simulink model "traal"  (R2019b)
settings: Solver=ode3  StartTime=0.0  StopTime=inf  RelTol=1e-3  EnableMultiTasking=on
undefined symbols (not defined in the file): Dist, Dist2, Ovrsht, Saved, trees
libraries: legoev3lib x15
settings Model: FPTRunName=Active  ExtModeTrigDuration=2  Creator=maarten  LastModifiedBy=Mohammed
settings SolverCC: PositivePriorityOrder=on
settings DataIOCC: LimitDataPoints=on  SaveFormat=Array
settings OptimizationCC: ExpressionDepthLimit=2147483647  LifeSpan=Inf  MaxStackSize=64
settings DebuggingCC: UnderspecifiedInitializationDetection=Classic  MergeDetectMultiDrivingBlocksExec=none  FcnCallInpInsideContextMsg=warning  AllowSymbolicDim=off  StateNameClashWarn=warning  SFUnexpectedBacktrackingDiag=warning  SFNoUnconditionalDefaultTransitionDiag=warning  SFExecutionAtInitializationDiag=none  ArithmeticOperatorsInVariantConditions=warning
settings HardwareCC: ProdBitPerPointer=32  ProdBitPerSizeT=32  ProdBitPerPtrDiffT=32  ProdLargestAtomicInteger=Long  ProdWordSize=32  ProdHWDeviceType=ARM Compatible->ARM 9  UseEmbeddedCoderFeatures=off  UseSimulinkCoderFeatures=off
settings ModelReferenceCC: PropagateSignalLabelsOutOfModel=off
settings SFSimCC: SimUseLocalCustomCode=off  CustomCodeUndefinedFunction=UseInterfaceOnly
settings RTWCC: SystemTargetFile=ert.tlc  HardwareBoard=LEGO MINDSTORMS EV3  TemplateMakefile=ert_default_tmf  GenerateReport=on  RTWVerbose=off  RTWUseLocalCustomCode=off  Toolchain=Sourcery G++ Lite v2009q3  BuildConfiguration=Faster Runs  LaunchReport=on
settings CodeAppCC: ForceParamTrailComments=on  OperatorAnnotations=on  MangleLength=10  StateflowObjectComments=on  MATLABSourceComments=on
settings ERTTargetCC: MultiwordLength=2048  ERTCustomFileBanners=off  SupportContinuousTime=on  SupportNonInlinedSFcns=on  RemoveResetFunc=off  SupportVariableSizeSignals=on  ModelStepFunctionPrototypeControlCompliant=off
settings ConfigComp: CovMetricSettings=dw  CovHtmlReporting=on  CovSaveCumulativeToWorkspaceVar=on  CovSaveSingleToWorkspaceVar=on  CovExternalEMLEnable=off  CovSFcnEnable=off

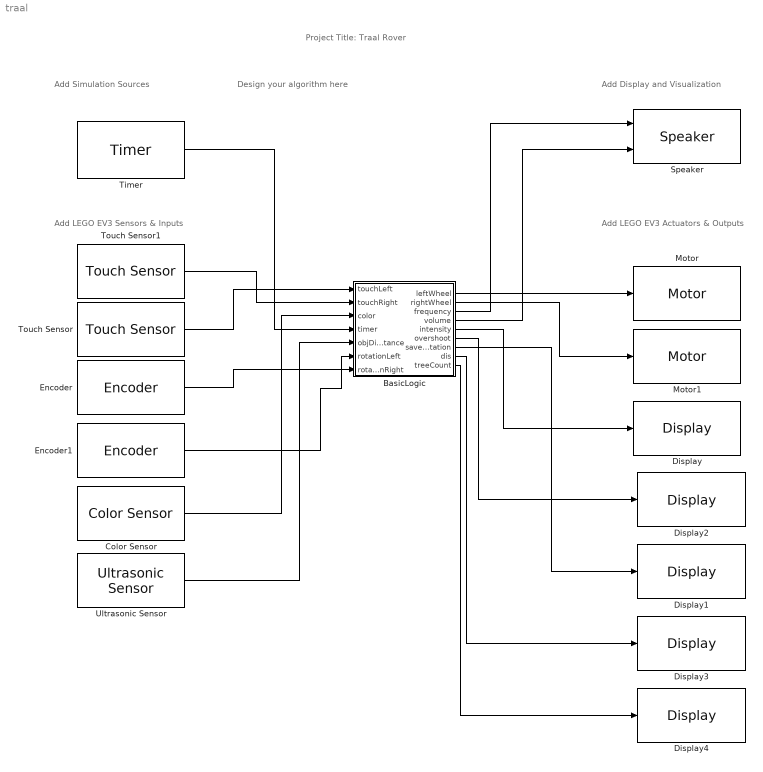
== system traal ==
  note: Project Title: Traal Rover
  note: Add LEGO EV3 Sensors & Inputs
  note: Add LEGO EV3 Actuators & Outputs
  note: Add Display and Visualization
  note: Design your algorithm here
  note: Add Simulation Sources
  BasicLogic : Stateflow chart  BlockKeywords=__PRM__SERIALIZED__DATA__:Stateflow Chart,Stateflow Diagram  TreatAsAtomicUnit=on
  Color Sensor : legoev3lib/Color Sensor  portNumber=3  mode=Reflected light intensity  sampleTime=0.1
      settings: SourceProductName=Simulink Support Package for LEGO MINDSTORMS EV3 Hardware  SourceProductBaseCode=LEGOEV3
  Display : legoev3lib/Display  slcdStr=Dist:  slcdLine=1  slcdFormat=Decimal
      settings: SourceProductName=Simulink Support Package for LEGO MINDSTORMS EV3 Hardware  SourceProductBaseCode=LEGOEV3
  Display1 : legoev3lib/Display  slcdStr=Saved:  slcdLine=3  slcdFormat=Decimal
      settings: SourceProductName=Simulink Support Package for LEGO MINDSTORMS EV3 Hardware  SourceProductBaseCode=LEGOEV3
  Display2 : legoev3lib/Display  slcdStr=Ovrsht:  slcdLine=2  slcdFormat=Decimal
      settings: SourceProductName=Simulink Support Package for LEGO MINDSTORMS EV3 Hardware  SourceProductBaseCode=LEGOEV3
  Display3 : legoev3lib/Display  slcdStr=Dist2:  slcdLine=4  slcdFormat=Decimal
      settings: SourceProductName=Simulink Support Package for LEGO MINDSTORMS EV3 Hardware  SourceProductBaseCode=LEGOEV3
  Display4 : legoev3lib/Display  slcdStr=trees:  slcdLine=5  slcdFormat=Decimal
      settings: SourceProductName=Simulink Support Package for LEGO MINDSTORMS EV3 Hardware  SourceProductBaseCode=LEGOEV3
  Encoder : legoev3lib/Encoder  portNumber=B  opMode=Reset by external signal  sampleTime=0.1
      settings: SourceProductName=Simulink Support Package for LEGO MINDSTORMS EV3 Hardware  SourceProductBaseCode=LEGOEV3
  Encoder1 : legoev3lib/Encoder  portNumber=C  opMode=Reset by external signal  sampleTime=0.1
      settings: SourceProductName=Simulink Support Package for LEGO MINDSTORMS EV3 Hardware  SourceProductBaseCode=LEGOEV3
  Motor : legoev3lib/Motor  sportNumber=C  sstopAction=Brake
  Motor1 : legoev3lib/Motor  sportNumber=B  sstopAction=Brake
  Speaker : legoev3lib/Speaker  sinputMode=Frequency and volume  sspeakerFreq=100  sspeakerVolume=50  sspeakerDuration=100
      settings: SourceProductName=Simulink Support Package for LEGO MINDSTORMS EV3 Hardware  SourceProductBaseCode=LEGOEV3
  Timer : legoev3lib/Timer  SampleTime=0.1
      settings: SourceProductName=Simulink Support Package for LEGO MINDSTORMS EV3 Hardware  SourceProductBaseCode=LEGOEV3
  Touch Sensor : legoev3lib/Touch Sensor  portNumber=1  sampleTime=0.1
      settings: SourceProductName=Simulink Support Package for LEGO MINDSTORMS EV3 Hardware  SourceProductBaseCode=LEGOEV3
  Touch Sensor1 : legoev3lib/Touch Sensor  portNumber=2  sampleTime=0.1
      settings: SourceProductName=Simulink Support Package for LEGO MINDSTORMS EV3 Hardware  SourceProductBaseCode=LEGOEV3
  Ultrasonic Sensor : legoev3lib/Ultrasonic Sensor  PortNumber=4  sampleTime=0.1
      settings: SourceProductName=Simulink Support Package for LEGO MINDSTORMS EV3 Hardware  SourceProductBaseCode=LEGOEV3
  wires:
  Touch Sensor/1 -> BasicLogic/1(touchLeft)
  BasicLogic/1(leftWheel) -> Motor/1
  BasicLogic/2(rightWheel) -> Motor1/1
  Touch Sensor1/1 -> BasicLogic/2(touchRight)
  Color Sensor/1 -> BasicLogic/3(color)
  Timer/1 -> BasicLogic/4(timer)
  BasicLogic/3(frequency) -> Speaker/1
  BasicLogic/4(volume) -> Speaker/2
  Ultrasonic Sensor/1 -> BasicLogic/5(objDistance)
  BasicLogic/5(intensity) -> Display/1
  Encoder/1 -> BasicLogic/7(rotationRight)
  Encoder1/1 -> BasicLogic/6(rotationLeft)
  BasicLogic/6(overshoot) -> Display2/1
  BasicLogic/7(savedRotation) -> Display1/1
  BasicLogic/8(dis) -> Display3/1
  BasicLogic/9(treeCount) -> Display4/1

== stateflow chart traal/BasicLogic ==
  state Master
    during:
    intensity = objDistance
    state ManualDriving
      during:
      dis = objDistance;
      state BothButtonsPressed
        entry:
        pressedTimer = timer
      state Forward
        entry: leftWheel = baseSpeed;
        rightWheel = baseSpeed;
        isStationary = false;
        fromAutonomous = false
      state Stationary
        entry: leftWheel = 0;
        rightWheel = 0;
        isStationary = true;
        fromAutonomous = false
      state ButtonsReleased
      state TurnLeft
        entry: leftWheel = 0;
        rightWheel = baseSpeed;
      state TurnRight
        entry: leftWheel = baseSpeed;
        rightWheel = 0;
      Forward -> (junction 31) [order 1] : [duration(touchLeft == 1) > 0.1]
      (default) -> Stationary
      Stationary -> BothButtonsPressed [order 3] : [touchLeft==1 && touchRight==1]
      Forward -> BothButtonsPressed [order 3] : [touchLeft==1 && touchRight==1]
      (junction 45) -> BothButtonsPressed : {isStationary = ~isStationary}
      BothButtonsPressed -> ButtonsReleased : [touchLeft==0 || touchRight==0]
      ButtonsReleased -> Stationary [order 3]
      ButtonsReleased -> Forward [order 2] : [timer - pressedTimer <= 1000 && isStationary]
      Stationary -> (junction 31) [order 2] : [duration(touchLeft == 1) > 0.2]
      (junction 31) -> TurnLeft
      Forward -> (junction 37) [order 2] : [duration(touchRight == 1) > 0.1]
      Stationary -> (junction 37) [order 1] : [duration(touchRight == 1) > 0.2]
      (junction 37) -> TurnRight
      TurnLeft -> (junction 45) : [touchLeft==0]
      TurnRight -> (junction 45) : [touchRight==0]
    state Finished
      entry:
      leftWheel = 0;
      rightWheel = 0;
      frequency = 4000;
      volume = 30;
      exit:
      frequency = 0;
      volume = 0;
    state Autonomous
      state GoToLine
        state goForward
          entry: leftWheel = 2 * baseSpeed;
          rightWheel = 2 * baseSpeed;
        state onLine
          entry:
          leftWheel = baseSpeed;
          rightWheel = baseSpeed;
        state BeyondLine
          entry: leftWheel = 0;
          rightWheel = 1.5 * baseSpeed;
        (default) -> goForward
        goForward -> onLine : [color < 25 ]
        onLine -> BeyondLine : [color > 20]
      state FollowLine
        during: dis = objDistance;
        state OnLine
          leftWheel = 1.5 * baseSpeed
          rightWheel = 1.5 * baseSpeed
          time = 0
        state startOnLine
          entry:
          leftWheel = baseSpeed
          rightWheel = baseSpeed
        state OffLineL
          entry:
          rightWheel = 1.5 * baseSpeed;
          leftWheel = - 1.5 * baseSpeed;
          time = time + 1;
        state OffLineR
          entry:
          leftWheel = 1.5 * baseSpeed;
          rightWheel = - 1.5 * baseSpeed;
          time = time + 1;
        (default) -> startOnLine
        OnLine -> OnLine [order 4] : [after(0.1,sec)]{counter = counter + 1}
        OnLine -> OffLineR [order 2] : [color > 20]
        OnLine -> OffLineL [order 1] : [color>20]
        OffLineL -> OnLine [order 1] : [color < 20]
        OffLineR -> OnLine [order 2] : [color < 20]
        startOnLine -> OffLineL : [color > 20]
        OffLineR -> OffLineL [order 1] : after(time,sec)
        OffLineL -> OffLineR [order 2] : after(time,sec)
      state AvoidObstacle
        state periodicLooking
          state turnLeft
            entry:
            leftWheel = -baseSpeed;
            rightWheel = baseSpeed;
            savedRotation = rotationLeft;
          state turnRight
            entry:
            leftWheel = baseSpeed;
            rightWheel = -baseSpeed;
            savedRotation = rotationRight;
          state driveStraight
            entry:
            leftWheel = baseSpeed;
            rightWheel = baseSpeed;
          state adjustLeft
            entry:
            leftWheel = -baseSpeed;
            rightWheel = baseSpeed;
            overshoot =  abs(savedRotation - rotationLeft) - degree90
            savedRotation = rotationLeft
            amountRightTurns = amountRightTurns + 1;
          (default) -> Master.Autonomous.AvoidObstacle.periodicLooking.turnLeft
          Master.Autonomous.AvoidObstacle.periodicLooking.turnRight -> Master.Autonomous.AvoidObstacle.periodicLooking.turnLeft [order 1] : [true == false]
          Master.Autonomous.AvoidObstacle.periodicLooking.turnLeft -> driveStraight : [abs(savedRotation - rotationLeft) > 160]
          driveStraight -> Master.Autonomous.AvoidObstacle.periodicLooking.turnRight : [after(2, sec)]
          Master.Autonomous.AvoidObstacle.periodicLooking.turnRight -> adjustLeft [order 2] : [objDistance > minObjDistanceT && rotationRight - savedRotation > 250 ]
          adjustLeft -> driveStraight : [abs(savedRotation - rotationLeft) > overshoot]
        state backWards
          entry:
          leftWheel = -baseSpeed
          rightWheel = -baseSpeed
        (default) -> backWards
        backWards -> periodicLooking : [after(1, sec)]
      state countTree
        state turnRight
          entry:
          leftWheel = baseSpeed;
          rightWheel = -baseSpeed;
          savedRotation = rotationRight;
          counter = 0;
        state turnLeft
          entry:
          leftWheel = -baseSpeed;
          rightWheel = baseSpeed;
          savedRotation = rotationLeft;
        (default) -> Master.Autonomous.countTree.turnRight
        Master.Autonomous.countTree.turnRight -> Master.Autonomous.countTree.turnLeft [order 1] : [(abs(savedRotation - rotationRight) > 130) && (objDistance < 50 ) && (objDistance > 15)]{treeCount = treeCount + 1 ; counter = -20}
        Master.Autonomous.countTree.turnRight -> Master.Autonomous.countTree.turnLeft [order 2] : [(abs(savedRotation - rotationRight) > 130) && not( (objDistance < 50 ) && (objDistance > 15) )]
      Master.Autonomous.countTree.turnLeft -> OnLine : [ (abs(savedRotation - rotationLeft) > 75)]
      OnLine -> countTree [order 3] : [counter == 5]
      BeyondLine -> FollowLine : [color < 20]
      (default) -> GoToLine
      AvoidObstacle -> GoToLine : [amountRightTurns > 5 && color < 20]{amountRightTurns = 0}
      GoToLine -> (junction 190) : [objDistance < 15]
      FollowLine -> (junction 190) : [objDistance < 15]
      (junction 190) -> AvoidObstacle
    (junction 150) -> (junction 45) : {fromAutonomous = true}
    (default) -> ManualDriving
    ButtonsReleased -> Autonomous [order 1] : [timer - pressedTimer > 1000 && ~fromAutonomous]
    Finished -> (junction 150) : [[duration(touchLeft==1) > 1.0 && duration(touchRight==1) > 1.0]]
    Autonomous -> (junction 150) [order 1] : [duration(touchLeft==1) > 1.0 && duration(touchRight==1) > 1.0]
    Autonomous -> Finished [order 2] : [color == 150]
  data: leftWheel output; rightWheel output; isStationary local =true; touchLeft input; touchRight input; baseSpeed constant double =20; color input; timer input; pressedTimer local; frequency output; volume output; objDistance input; intensity output; time local =0; rotationLeft input; rotationRight input; amountRightTurns local =0; minObjDistanceT local =30; overshoot output; degree90 local =90; savedRotation output; fromAutonomous local =false; dis output; counter local =3; treeCount output =0
